simulink model "Quadcopter_LQR_PI_Observer_3DOF"  (R2022a)
settings: Solver=VariableStepAuto  StartTime=0.0  StopTime=10.0  RelTol=1e-3
undefined symbols (not defined in the file): A, B, C, Klqr, L
settings Model: Creator=creec  LastModifiedBy=creec

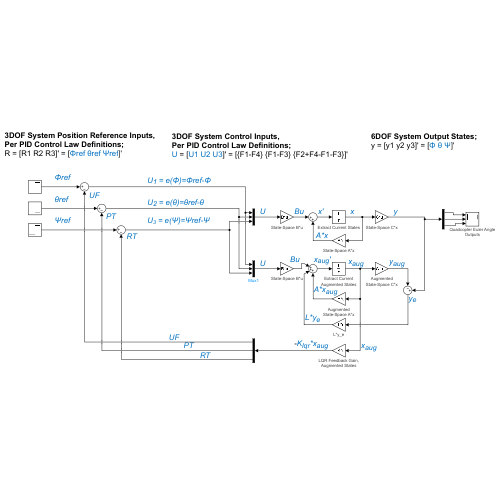
[thumbnail: Simulink's stored preview of the top-level diagram]
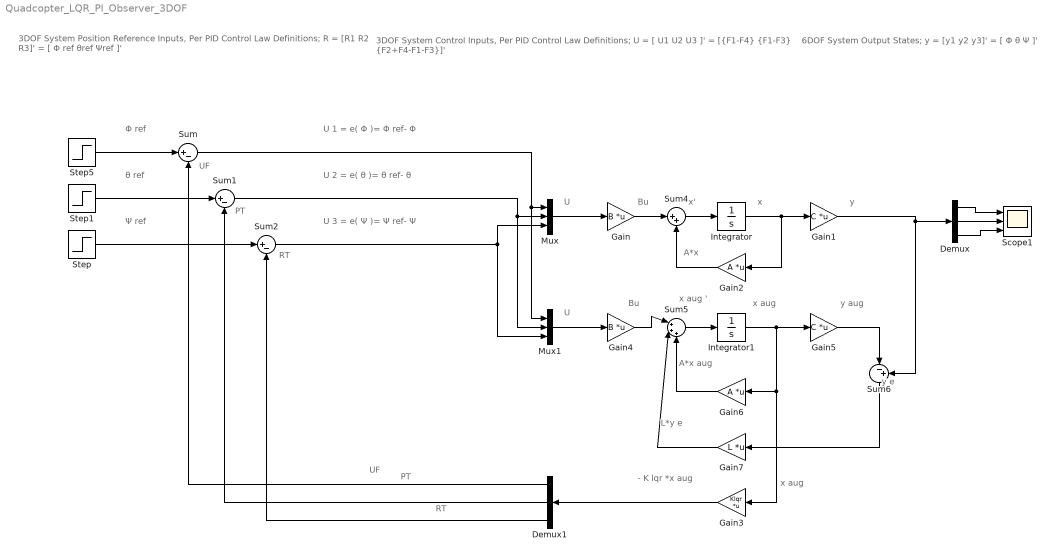
== system Quadcopter_LQR_PI_Observer_3DOF ==
  note: U 3 = e( Ψ )= Ψ ref- Ψ
  note: U 2 = e( θ )= θ ref- θ
  note: Bu
  note: 3DOF System Position Reference Inputs,
      | Per PID Control Law Definitions;
      | R = [R1 R2 R3]' = [ Φ ref θref Ψref ]'
  note: - K lqr *x aug
  note: UF
  note: U 1 = e( Φ )= Φ ref- Φ
  note: PT
  note: RT
  note: Φ ref
  note: y
  note: θ ref
  note: PT
  note: A*x
  note: x
  note: UF
  note: RT
  note: x aug
  note: Bu
  note: 6DOF System Output States;
      | y = [y1 y2 y3]' = [ Φ θ Ψ ]'
  note: y aug
  note: x'
  note: 3DOF System Control Inputs,
      | Per PID Control Law Definitions;
      | U = [ U1 U2 U3 ]' = [{F1-F4} {F1-F3} {F2+F4-F1-F3}]'
  note: y e
  note: A*x aug
  note: Ψ ref
  note: x aug
  note: x aug '
  note: U
  note: U
  note: L*y e
  Demux : Demux  Outputs=3
  Demux1 : Demux  Outputs=3
  Gain : Gain  Gain=B  Multiplication=Matrix(K*u)
      settings: AttributesFormatString=State-Space B*u
  Gain1 : Gain  Gain=C  Multiplication=Matrix(K*u)
      settings: AttributesFormatString=State-Space C*x
  Gain2 : Gain  Gain=A  Multiplication=Matrix(K*u)
      settings: AttributesFormatString=State-Space A*x
  Gain3 : Gain  Gain=Klqr  Multiplication=Matrix(K*u)
      settings: AttributesFormatString=|
      | LQR Feedback Gain,
      | Augmented States
  Gain4 : Gain  Gain=B  Multiplication=Matrix(K*u)
      settings: AttributesFormatString=State-Space B*u
  Gain5 : Gain  Gain=C  Multiplication=Matrix(K*u)
      settings: AttributesFormatString=|
      | Augmented
      | State-Space C*x
  Gain6 : Gain  Gain=A  Multiplication=Matrix(K*u)
      settings: AttributesFormatString=|
      | Augmented
      | State-Space A*x
  Gain7 : Gain  Gain=L  Multiplication=Matrix(K*u)
      settings: AttributesFormatString=L*y_e
  Integrator : Integrator
      settings: AttributesFormatString=Extract Current States
  Integrator1 : Integrator
      settings: AttributesFormatString=|
      | Extract Current
      | Augmented States
  Mux : Mux  Inputs=3
  Mux1 : Mux  Inputs=3
  Scope1 : Scope  NumInputPorts=3
      settings: AttributesFormatString=|
      | Quadcopter Euler Angle
      | Outputs
  Step : Step  After=1.5  SampleTime=0
  Step1 : Step  After=-2  SampleTime=0
  Step5 : Step  SampleTime=0
  Sum : Sum  Inputs=|+-
  Sum1 : Sum  Inputs=|+-
  Sum2 : Sum  Inputs=|+-
  Sum4 : Sum  Inputs=|++
  Sum5 : Sum  Inputs=|+++
  Sum6 : Sum  Inputs=|-+
  wires:
  Integrator1/1 -> Gain3/1, Gain6/1, Gain5/1
  Sum6/1 -> Gain7/1
  Sum5/1 -> Integrator1/1
  Gain1/1 -> Sum6/2, Demux/1
  Mux/1 -> Gain/1
  Sum2/1 -> Mux/3, Mux1/3
  Sum4/1 -> Integrator/1
  Integrator/1 -> Gain2/1, Gain1/1
  Sum/1 -> Mux1/1, Mux/1
  Step5/1 -> Sum/1
  Gain7/1 -> Sum5/2
  Mux1/1 -> Gain4/1
  Gain2/1 -> Sum4/2
  Step/1 -> Sum2/1
  Demux1/1 -> Sum/2
  Gain/1 -> Sum4/1
  Demux1/2 -> Sum1/2
  Gain3/1 -> Demux1/1
  Gain5/1 -> Sum6/1
  Sum1/1 -> Mux/2, Mux1/2
  Demux1/3 -> Sum2/2
  Gain6/1 -> Sum5/3
  Gain4/1 -> Sum5/1
  Step1/1 -> Sum1/1
  Demux/1 -> Scope1/1
  Demux/2 -> Scope1/2
  Demux/3 -> Scope1/3
